simulink model "gm_tmod"  (R2018a)
settings: Solver=FixedStepAuto  StartTime=0.0  StopTime=0.2  RelTol=1e-3  EnableMultiTasking=on
libraries: simulink x1, dspsrcs4 x1
settings Model: Creator=klutc_000  LastModifiedBy=klutc_000
settings SolverCC: AutoInsertRateTranBlk=on
settings OptimizationCC: BlockReduction=off  ConditionallyExecuteInputs=off
settings DebuggingCC: InheritedTsInSrcMsg=none  SingleTaskRateTransMsg=error

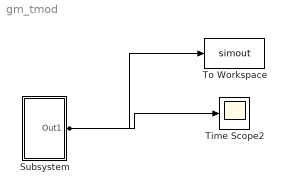
== system gm_tmod ==
  Subsystem : Subsystem
  Time Scope2 : Scope
  To Workspace : ToWorkspace  VariableName=simout  SampleTime=-1
  wires:
  Subsystem/1(Out1) -> Time Scope2/1, To Workspace/1

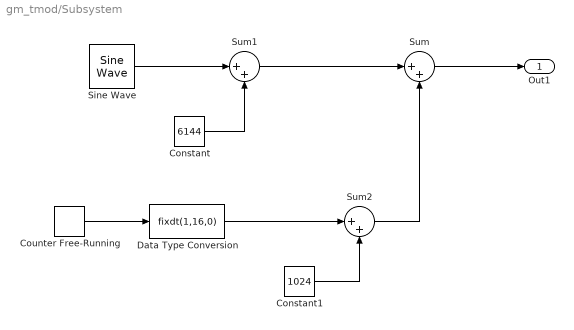
== system gm_tmod/Subsystem ==
  Constant : Constant  Value=6144  OutDataTypeStr=int16
  Constant1 : Constant  Value=1024  OutDataTypeStr=fixdt(1,16,0)
  Counter Free-Running : simulink/Sources/Counter Free-Running  NumBits=11  tsamp=1/10000
  Data Type Conversion : DataTypeConversion  OutMax=[1023]  OutDataTypeStr=fixdt(1,16,0)
  Sine Wave : dspsrcs4/Sine Wave  Amplitude=6143  Frequency=10  Phase=0  SampleMode=Discrete  OutComplex=Real  CompMethod=Table lookup  TableSize=Speed  SampleTime=1/10000  SamplesPerFrame=1  ResetState=Restart at time zero  OutputFrames=off  dataType=Fixed-point  wordLen=16  udDataType=sfix(16)  fracBitsMode=User-defined  numFracBits=0  OutDataTypeStr=fixdt(1,16,0)  LastOutDataTypeStr=fixdt(1,16,0)
  Sum : Sum  Inputs=|++  OutMin=[0]  OutMax=[16383]  OutDataTypeStr=uint16
  Sum1 : Sum  Inputs=|++  OutMin=[0]  OutMax=[16383]  OutDataTypeStr=fixdt(1,16,0)
  Sum2 : Sum  Inputs=|++  OutMin=[0]  OutMax=[16383]  OutDataTypeStr=fixdt(1,16,0)
  Out1 : Outport
  wires:
  Constant/1 -> Sum1/2
  Constant1/1 -> Sum2/2
  Counter Free-Running/1 -> Data Type Conversion/1
  Data Type Conversion/1 -> Sum2/1
  Sine Wave/1 -> Sum1/1
  Sum/1 -> Out1/1
  Sum1/1 -> Sum/1
  Sum2/1 -> Sum/2
